simulink model "BlackBird"  (R2024b)
settings: Solver=VariableStepAuto  StartTime=0.0  StopTime=tf  RelTol=1e-3
values from neighbouring files (symbols this model uses):
  alpha0__rad = 4*pi/180    (= 0.0698131700798)    [Main.m]
  beta0__rad = 0    [Main.m]
  cbar__m = ac.cbar__m    [ComputePitchRates.m]    (also in Main.m = cbar__ft * 0.3048)
  del_ail__rad = 0.3 * pi/180    (= 0.00523598775598)    [Main.m]
  inertia_tensor = [Ixx__kgm2, 0,-Ixz__kgm2 ... (first row only)    [Main.m]
  mass__kg = mass__lb * 0.224808943    [Main.m]
  max_thrust_unit__N = max_thrust_unit__lbf * 4.448    [Main.m]
  p0__rad_s = 0    [Main.m]
  phi0__rad = 0    [Main.m]
  psi0__rad = 0    [Main.m]
  q0__rad_s = 0    [Main.m]
  r0__rad_s = 0    [Main.m]
  theta0__rad = 0    [Main.m]
  throttle = 0.1072    [Main.m]
  u0__m_s = 600    [Main.m]
  v0__m_s = 0    [Main.m]
  w0__m_s = 0    [Main.m]
  wingarea__m2 = ac.wingarea__m2    [ComputePitchRates.m]    (also in ComputeRollYawRates.m; Main.m = wingarea__ft2 * 0.09290304)
  wingspan__m = ac.wingspan__m    [ComputeRollYawRates.m]    (also in Main.m = wingspan__ft * 0.3048)
  x0__m = 0    [Main.m]
  y0__m = 0    [Main.m]
  z0__m = -20000    [Main.m]
undefined symbols (not defined in the file or in its folder): A, Blackbird, CD_f, cL0_f, cl0_m, cLalpha_f__deg, clbeta_m__deg, cLdelta_f_e__deg, cldelta_m_a__deg, cldelta_m_r__deg, clp_m__rad, cLq_f__rad, clr_m__rad, cm0_m, cmalpha_m__deg, cmdelta_m_e__deg, cmq_m__rad, cn0_m, cnbeta_m__deg, cndelta_m_a__deg, cndelta_m_r__deg, cnp_m__rad, cnr_m__rad, cY0_f, cYbeta_f__deg, cYdelta_f_a__deg, cYdelta_f_r__deg, cYp_f__rad, cYr_f__rad, Earth, WGS84
libraries: simulink_extras x25, aerolibfltsims x2, simulink x2, aerolibtransform2 x1, aerolibatmos2 x1, matrix_library x1
settings Model: Creator=alexa  LastModifiedBy=alexa
settings SolverCC: AlgebraicLoopSolver=TrustRegion
settings SFSimCC: CustomCodeUndefinedFunction=UseInterfaceOnly
settings RTWCC: GPUComputeCapability=3.5

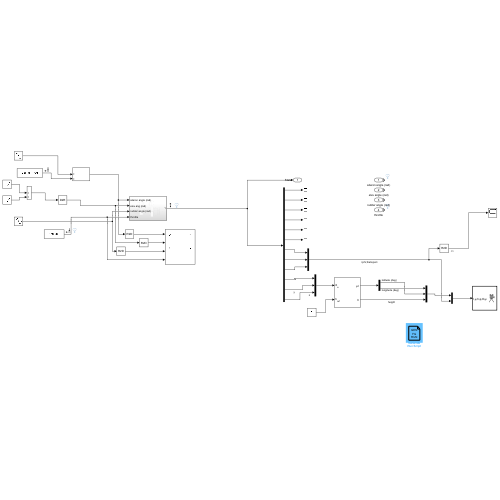
[thumbnail: Simulink's stored preview of the top-level diagram]
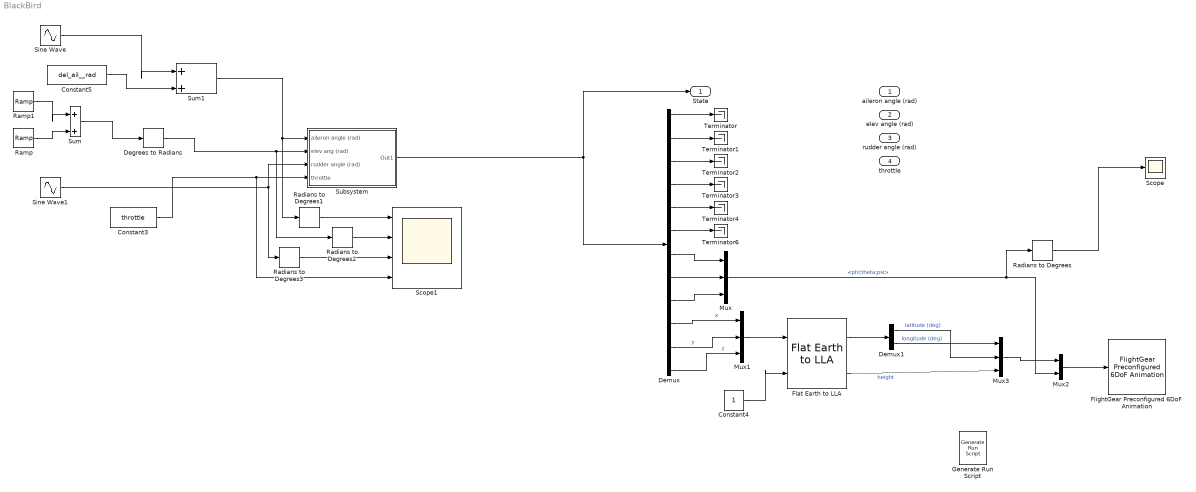
== system BlackBird ==
  aileron angle (rad) : Inport
  elev angle (rad) : Inport  Port=2
  rudder angle (rad) : Inport  Port=3
  throttle : Inport  Port=4
  Constant3 : Constant  Value=throttle
  Constant4 : Constant
  Constant5 : Constant  Value=del_ail__rad
  Degrees to Radians : simulink_extras/Transformations/Degrees to Radians
  Demux : Demux  Outputs=12
  Demux1 : Demux  Outputs=2
  Flat Earth to LLA : aerolibtransform2/Flat Earth to LLA  units=Metric (MKS)  ptype=Earth (WGS84)  F=1/298.257223563  R=6378137  refPosPort=off  LL0=[0 10]  psi=0
  FlightGear Preconfigured 6DoF Animation : aerolibfltsims/FlightGear Preconfigured 6DoF Animation  xFlightGearVersion=v2019.1  DestinationIpAddress=127.0.0.1  DestinationPort=5502  SampleTime=1/30  packetVersion=24
  Generate Run Script : aerolibfltsims/Generate Run Script  Architecture=Win64  dataFlow=Send  GeometryModelName=Blackbird-A  AirportId=KSFO  RunwayId=10L  InitialAltitude=7224  InitialHeading=113  OffsetDistance=4.72  OffsetAzimuth=0  InstallScenery=off  DisableShaders=on  OriginAddress=127.0.0.1  DestinationPort=5502  OriginPort=5505  LocalAddress=127.0.0.1  OutputFileName=runfg.bat  FlightGearBaseDirectory=C:\Program Files\FlightGear 2020.3
  Mux : Mux  Inputs=3
  Mux1 : Mux  Inputs=3
  Mux2 : Mux  Inputs=2
  Mux3 : Mux  Inputs=3
  Radians to Degrees{,1..3} (4 alike) : simulink_extras/Transformations/Radians to Degrees
  Ramp : simulink/Sources/Ramp  slope=-1  start=0  InitialOutput=0
  Ramp1 : simulink/Sources/Ramp  slope=2  start=14  InitialOutput=0
  Scope : Scope
  Scope1 : Scope  NumInputPorts=4
  Sine Wave : Sin  Amplitude=3*pi/180  Frequency=0.3  SampleTime=0
  Sine Wave1 : Sin  Amplitude=1.5*pi/180  Frequency=0.3  SampleTime=0
  Subsystem : Subsystem
  Sum : Sum  Inputs=|++
  Sum1 : Sum  Inputs=|++
  Terminator{,1..4,6} (6 alike) : Terminator
  State : Outport
  wires:
  Sum1/1 -> Radians to Degrees1/1, Subsystem/1(aileron angle (rad))
  Degrees to Radians/1 -> Radians to Degrees2/1, Subsystem/2(elev ang (rad))
  Sine Wave1/1 -> Subsystem/3(rudder angle (rad)), Radians to Degrees3/1
  Constant3/1 -> Scope1/4, Subsystem/4(throttle)
  Subsystem/1(Out1) -> Demux/1, State/1
  Demux/1 -> Terminator/1
  Demux/2 -> Terminator1/1
  Demux/3 -> Terminator2/1
  Demux/4 -> Terminator3/1
  Demux/5 -> Terminator4/1
  Demux/6 -> Terminator6/1
  Demux/7 -> Mux/1
  Demux/8 -> Mux/2
  Demux/9 -> Mux/3
  Demux/10 -> Mux1/1  "x"
  Demux/11 -> Mux1/2  "y"
  Mux/1 -> Radians to Degrees/1, Mux2/2  "<phi;theta;psi>"
  Mux2/1 -> FlightGear Preconfigured 6DoF Animation/1
  Demux/12 -> Mux1/3  "z"
  Mux1/1 -> Flat Earth to LLA/1
  Flat Earth to LLA/1 -> Demux1/1
  Demux1/1 -> Mux3/2  "latitude (deg)"
  Demux1/2 -> Mux3/1  "longitude (deg)"
  Flat Earth to LLA/2 -> Mux3/3  "height"
  Mux3/1 -> Mux2/1
  Constant4/1 -> Flat Earth to LLA/2
  Sum/1 -> Degrees to Radians/1
  Ramp/1 -> Sum/2
  Ramp1/1 -> Sum/1
  Radians to Degrees/1 -> Scope/1
  Radians to Degrees1/1 -> Scope1/1
  Radians to Degrees2/1 -> Scope1/2
  Radians to Degrees3/1 -> Scope1/3
  Sine Wave/1 -> Sum1/1
  Constant5/1 -> Sum1/2

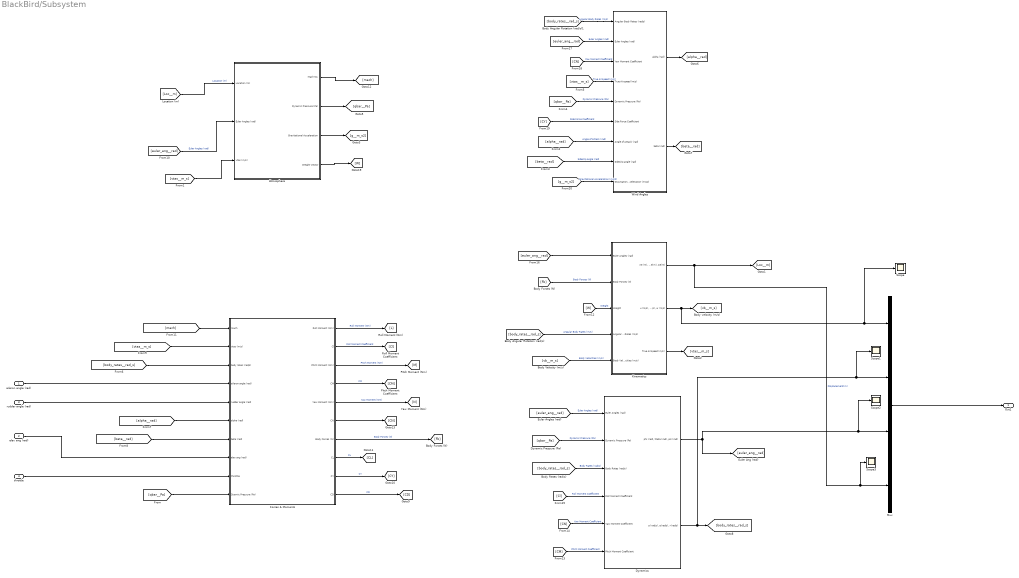
== system BlackBird/Subsystem ==
  aileron angle (rad) : Inport
  elev ang (rad) : Inport  Port=2
  rudder angle (rad) : Inport  Port=3
  throttle : Inport  Port=4
  Atmosphere : Subsystem
  Dynamics : Subsystem
  Forces & Moments : Subsystem
  Kinematics : Subsystem
  Mux : Mux
  Scope{,1..3} (4 alike) : Scope
  Wind Angles : Subsystem
  Out1 : Outport
  wires:
  Forces & Moments/9(CY) -> [CY]  "CY"
  Dynamics/2("p (rad/s), q(rad/s), r(rad/s)") -> Scope1/1, Mux/2, [body_rates__rad_s]
  [euler_ang__rad] -> Atmosphere/2(Euler Angles (rad))  "Euler Angles (rad)"
  [CM] -> Dynamics/6(Pitch Moment Coefficient)  "Pitch Moment Coefficient"
  Forces & Moments/4(CM) -> [CM]  "CM"
  [alpha__rad] -> Forces & Moments/6(alpha (rad))
  Forces & Moments/10(CD) -> [CD]  "CD"
  [mach] -> Forces & Moments/1(mach)
  [Fb] -> Kinematics/2(Body Forces (N))  "Body Forces (N)"
  Mux/1 -> Out1/1
  [W] -> Kinematics/3(Weight)  "Weight"
  Wind Angles/1(alpha (rad)) -> [alpha__rad]
  elev ang (rad)/1 -> Forces & Moments/8(elev ang (rad))
  Dynamics/1("phi (rad), theta (rad), psi (rad)") -> Scope2/1, Mux/3, [euler_ang__rad]
  [beta__rad] -> Forces & Moments/7(beta (rad))
  [euler_ang__rad] -> Wind Angles/2(Euler Angles (rad))  "Euler Angles (rad)"
  [euler_ang__rad] -> Kinematics/1(Euler Angles (rad))
  [euler_ang__rad] -> Dynamics/1(Euler Angles (rad))  "Euler Angles (rad)"
  Forces & Moments/2(Cl) -> [Cl]  "Roll Moment Coefficient"
  Kinematics/1("Xe (m), Ye(m), Ze(m)") -> [Loc__m], Scope3/1, Mux/4  "Displacement(m)"
  Forces & Moments/7(Body Forces (N)) -> [Fb]  "Body Forces (N)"
  Atmosphere/1(Mach No.) -> [mach]
  Forces & Moments/6(CN) -> [CN]
  [body_rates__rad_s] -> Forces & Moments/3(body rates (rad/s))
  [body_rates__rad_s] -> Wind Angles/1(Angular Body Rates (rad/s))  "Angular Body Rates (m/s)"
  [qbar__Pa] -> Dynamics/2(Dynamic Pressure (Pa))  "Dynamic Pressure (Pa)"
  Forces & Moments/3(Pitch Moment (Nm)) -> [M]  "Pitch Moment (Nm)"
  [vtas__m_s] -> Forces & Moments/2(vtas (m/s))
  Forces & Moments/1(Roll Moment (Nm)) -> [L]  "Roll Moment (Nm)"
  Kinematics/2("u (m/s), v(m/s), w (m/s)") -> Scope/1, Mux/1, [vb__m_s]
  Kinematics/3(True Airspeed (m/s)) -> [vtas__m_s]
  [beta__rad] -> Wind Angles/8(Sideslip angle (rad))  "Sideslip angle (rad)"
  [body_rates__rad_s] -> Dynamics/3(Body Rates (rad/s))  "Body Rates (rad/s)"
  rudder angle (rad)/1 -> Forces & Moments/5(rudder angle (rad))
  Forces & Moments/5(Yaw Moment (Nm)) -> [N]  "Yaw Moment (Nm)"
  Forces & Moments/8(CL) -> [CL]  "CL"
  [Cl] -> Dynamics/4(Roll Moment Coefficient)  "Roll Moment Coefficient"
  [CN] -> Wind Angles/3(Yaw Moment Coefficient)  "Yaw Moment Coefficient"
  Atmosphere/3(Gravitational Acceleration) -> [g__m_s2]
  [CN] -> Dynamics/5(Yaw Moment Coefficient)  "Yaw Moment Coefficient"
  [vb__m_s] -> Kinematics/5(Body Velocities (m/s))  "Body Velocities (m/s)"
  [Loc__m] -> Atmosphere/1(Location (m))  "Location (m)"
  Atmosphere/2(Dynamic Pressure (Pa)) -> [qbar__Pa]
  [qbar__Pa] -> Wind Angles/5(Dynamic Pressure (Pa))  "Dynamic Pressure (Pa)"
  Atmosphere/4(Weight Vector) -> [W]
  [body_rates__rad_s] -> Kinematics/4(Angular Body Rates (m/s))  "Angular Body Rates (m/s)"
  [alpha__rad] -> Wind Angles/7(Angle of Attack (rad))  "Angle of Attack (rad)"
  Wind Angles/2(beta (rad)) -> [beta__rad]
  [vtas__m_s] -> Wind Angles/4(True Airspeed (m/s))  "True Airspeed (m/s)"
  [g__m_s2] -> Wind Angles/9(Gravitational Acceleration (m/s2))  "Gravitational Acceleration (m/s2)"
  [CY] -> Wind Angles/6(Side Force Coefficient)  "Side Force Coefficient"
  throttle/1 -> Forces & Moments/9(throttle)
  aileron angle (rad)/1 -> Forces & Moments/4(aileron angle (rad))
  [qbar__Pa] -> Forces & Moments/10(Dyamic Pressure (Pa))
  [vtas__m_s] -> Atmosphere/3(vtas (m/s))

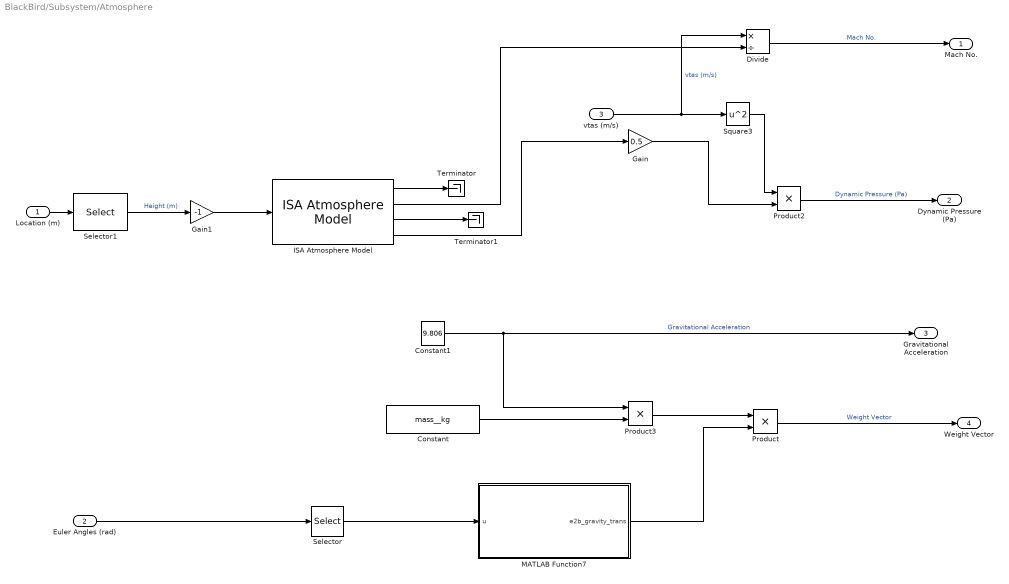
== system BlackBird/Subsystem/Atmosphere ==
  Location (m) : Inport
  Euler Angles (rad) : Inport  Port=2
  vtas (m/s) : Inport  Port=3
  Constant : Constant  Value=mass__kg
  Constant1 : Constant  Value=9.806
  Divide : Product  Inputs=*/
  Gain : Gain  Gain=0.5
  Gain1 : Gain  Gain=-1
  ISA Atmosphere Model : aerolibatmos2/ISA Atmosphere Model  useExtended=off  action=Warning  custom=off  viscosityOut=off  g=9.80665  gamma=1.4  R=287.0531  L=0.0065  h_trop=11000  h_strat=20000  rho0=1.225  P0=101325  T0=288.15  h0=0  S=110.4  Tref=273.15  muref=1.716e-5
  MATLAB Function7 : MATLAB Function  TreatAsAtomicUnit=on
  Product : Product
  Product2 : Product
  Product3 : Product
  Selector : Selector  InputPortWidth=3  IndexOptions=Index vector (dialog)  Indices=[1 2]  OutputSizes=1
  Selector1 : Selector  InputPortWidth=3  IndexOptions=Index vector (dialog)  Indices=[3]  OutputSizes=1
  Square3 : Math  Operator=square
  Terminator : Terminator
  Terminator1 : Terminator
  Mach No. : Outport
  Dynamic Pressure (Pa) : Outport  Port=2
  Gravitational Acceleration : Outport  Port=3
  Weight Vector : Outport  Port=4
  wires:
  Product3/1 -> Product/1
  ISA Atmosphere Model/1 -> Terminator/1
  Gain/1 -> Product2/2
  Constant1/1 -> Gravitational Acceleration/1, Product3/1  "Gravitational Acceleration"
  ISA Atmosphere Model/3 -> Terminator1/1
  Selector/1 -> MATLAB Function7/1(u)
  Square3/1 -> Product2/1
  ISA Atmosphere Model/4 -> Gain/1
  vtas (m/s)/1 -> Divide/1, Square3/1  "vtas (m/s)"
  MATLAB Function7/1(e2b_gravity_trans) -> Product/2
  ISA Atmosphere Model/2 -> Divide/2
  Constant/1 -> Product3/2
  Product/1 -> Weight Vector/1  "Weight Vector"
  Divide/1 -> Mach No./1  "Mach No."
  Product2/1 -> Dynamic Pressure (Pa)/1  "Dynamic Pressure (Pa)"
  Euler Angles (rad)/1 -> Selector/1
  Selector1/1 -> Gain1/1  "Height (m)"
  Location (m)/1 -> Selector1/1
  Gain1/1 -> ISA Atmosphere Model/1

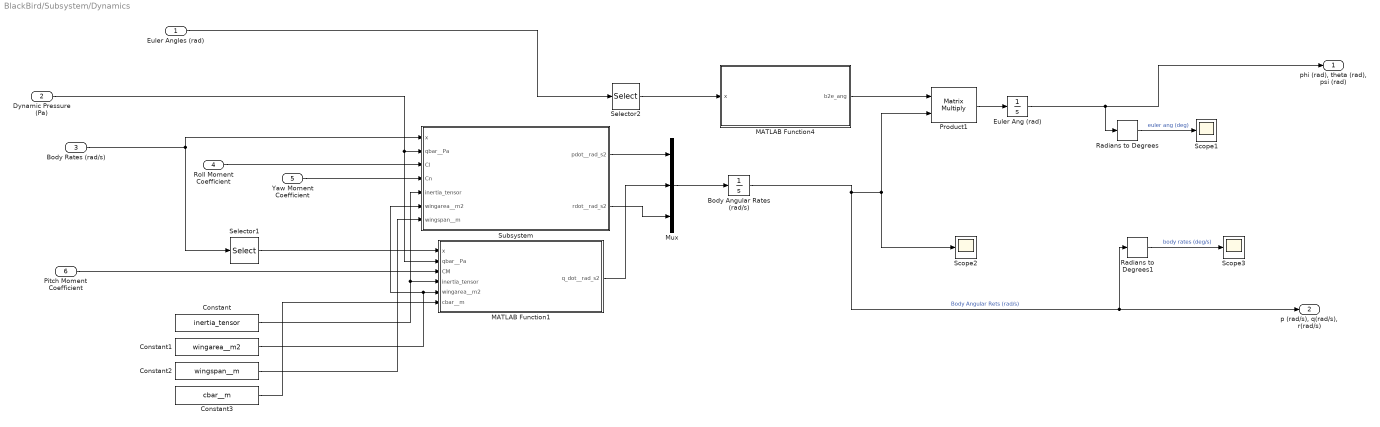
== system BlackBird/Subsystem/Dynamics ==
  Euler Angles (rad) : Inport
  Dynamic Pressure (Pa) : Inport  Port=2
  Body Rates (rad/s) : Inport  Port=3
  Roll Moment Coefficient : Inport  Port=4
  Yaw Moment Coefficient : Inport  Port=5
  Pitch Moment Coefficient : Inport  Port=6
  " Body Angular Rates (rad/s)" : Integrator  InitialCondition=[p0__rad_s;q0__rad_s;r0__rad_s]
  Constant : Constant  Value=inertia_tensor
  Constant1 : Constant  Value=wingarea__m2
  Constant2 : Constant  Value=wingspan__m
  Constant3 : Constant  Value=cbar__m
  Euler Ang (rad) : Integrator  InitialCondition=[phi0__rad;theta0__rad;psi0__rad]
  MATLAB Function1 : MATLAB Function  TreatAsAtomicUnit=on
  MATLAB Function4 : MATLAB Function  TreatAsAtomicUnit=on
  Mux : Mux  Inputs=3
  Product1 : Product  Multiplication=Matrix(*)
  Radians to Degrees : simulink_extras/Transformations/Radians to Degrees
  Radians to Degrees1 : simulink_extras/Transformations/Radians to Degrees
  Scope1 : Scope
  Scope2 : Scope
  Scope3 : Scope
  Selector1 : Selector  InputPortWidth=3  IndexOptions=Index vector (dialog)  Indices=[1 3]  OutputSizes=1
  Selector2 : Selector  InputPortWidth=3  IndexOptions=Index vector (dialog)  Indices=[1 2]  OutputSizes=1
  Subsystem : Subsystem
  "phi (rad), theta (rad), psi (rad)" : Outport
  "p (rad/s), q(rad/s), r(rad/s)" : Outport  Port=2
  wires:
  " Body Angular Rates (rad/s)"/1 -> Radians to Degrees1/1, "p (rad/s), q(rad/s), r(rad/s)"/1, Scope2/1, Product1/2  "Body Angular Rets (rad/s)"
  Dynamic Pressure (Pa)/1 -> MATLAB Function1/2(qbar__Pa), Subsystem/2(qbar__Pa)
  Selector1/1 -> MATLAB Function1/1(x)
  Product1/1 -> Euler Ang (rad)/1
  MATLAB Function4/1(b2e_ang) -> Product1/1
  Mux/1 -> " Body Angular Rates (rad/s)"/1
  Euler Ang (rad)/1 -> Radians to Degrees/1, "phi (rad), theta (rad), psi (rad)"/1
  MATLAB Function1/1(q_dot__rad_s2) -> Mux/2
  Selector2/1 -> MATLAB Function4/1(x)
  Pitch Moment Coefficient/1 -> MATLAB Function1/3(CM)
  Euler Angles (rad)/1 -> Selector2/1
  Constant/1 -> Subsystem/5(inertia_tensor), MATLAB Function1/4(inertia_tensor)
  Constant1/1 -> Subsystem/6(wingarea__m2), MATLAB Function1/5(wingarea__m2)
  Constant3/1 -> MATLAB Function1/6(cbar__m)
  Body Rates (rad/s)/1 -> Selector1/1, Subsystem/1(x)
  Roll Moment Coefficient/1 -> Subsystem/3(Cl)
  Yaw Moment Coefficient/1 -> Subsystem/4(Cn)
  Constant2/1 -> Subsystem/7(wingspan__m)
  Subsystem/1(pdot__rad_s2) -> Mux/1
  Subsystem/2(rdot__rad_s2) -> Mux/3
  Radians to Degrees/1 -> Scope1/1  "euler ang (deg)"
  Radians to Degrees1/1 -> Scope3/1  "body rates (deg/s)"

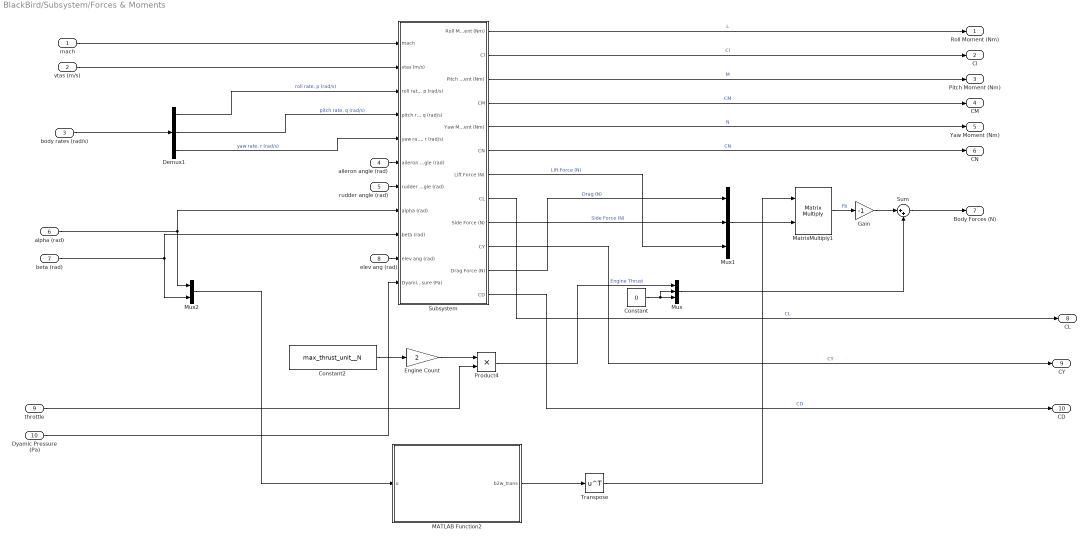
== system BlackBird/Subsystem/Forces & Moments ==
  mach : Inport
  vtas (m/s) : Inport  Port=2
  body rates (rad/s) : Inport  Port=3
  aileron angle (rad) : Inport  Port=4
  rudder angle (rad) : Inport  Port=5
  alpha (rad) : Inport  Port=6
  beta (rad) : Inport  Port=7
  elev ang (rad) : Inport  Port=8
  throttle : Inport  Port=9
  Dyamic Pressure (Pa) : Inport  Port=10
  Constant : Constant  Value=0
  Constant2 : Constant  Value=max_thrust_unit__N
  Demux1 : Demux  Outputs=3
  Engine Count : Gain  Gain=2
  Gain : Gain  Gain=-1
  MATLAB Function2 : MATLAB Function  TreatAsAtomicUnit=on
  MatrixMultiply1 : Product  Multiplication=Matrix(*)
  Mux : Mux  Inputs=3
  Mux1 : Mux  Inputs=3
  Mux2 : Mux  Inputs=2
  Product4 : Product
  Subsystem : Subsystem
  Sum : Sum  Inputs=|++
  Transpose : Math  Operator=transpose
  Roll Moment (Nm) : Outport
  Cl : Outport  Port=2
  Pitch Moment (Nm) : Outport  Port=3
  CM : Outport  Port=4
  Yaw Moment (Nm) : Outport  Port=5
  CN : Outport  Port=6
  Body Forces (N) : Outport  Port=7
  CL : Outport  Port=8
  CY : Outport  Port=9
  CD : Outport  Port=10
  wires:
  MATLAB Function2/1(b2w_trans) -> Transpose/1
  Constant2/1 -> Engine Count/1
  Transpose/1 -> MatrixMultiply1/1
  Subsystem/8(CL) -> CL/1  "CL"
  Demux1/1 -> Subsystem/3("roll rate, p (rad/s)")  "roll rate, p (rad/s)"
  throttle/1 -> Product4/2
  alpha (rad)/1 -> Mux2/1, Subsystem/8(alpha (rad))
  beta (rad)/1 -> Mux2/2, Subsystem/9(beta (rad))
  Subsystem/1(Roll Moment (Nm)) -> Roll Moment (Nm)/1  "L"
  Engine Count/1 -> Product4/1
  Subsystem/9(Side Force (N)) -> Mux1/2  "Side Force (N)"
  mach/1 -> Subsystem/1(mach)
  Mux1/1 -> MatrixMultiply1/2
  Subsystem/12(CD) -> CD/1  "CD"
  Subsystem/10(CY) -> CY/1  "CY"
  Demux1/3 -> Subsystem/5("yaw rate, r (rad/s)")  "yaw rate, r (rad/s)"
  Demux1/2 -> Subsystem/4("pitch rate, q (rad/s)")  "pitch rate, q (rad/s)"
  Subsystem/11(Drag Force (N)) -> Mux1/1  "Drag (N)"
  vtas (m/s)/1 -> Subsystem/2(vtas (m/s))
  Mux2/1 -> MATLAB Function2/1(u)
  Product4/1 -> Mux/1  "Engine Thrust"
  Subsystem/4(CM) -> CM/1  "CM"
  body rates (rad/s)/1 -> Demux1/1
  aileron angle (rad)/1 -> Subsystem/6(aileron angle (rad))
  Subsystem/3(Pitch Moment (Nm)) -> Pitch Moment (Nm)/1  "M"
  Subsystem/2(Cl) -> Cl/1  "Cl"
  rudder angle (rad)/1 -> Subsystem/7(rudder angle (rad))
  Subsystem/6(CN) -> CN/1  "CN"
  Subsystem/5(Yaw Moment (Nm)) -> Yaw Moment (Nm)/1  "N"
  elev ang (rad)/1 -> Subsystem/10(elev ang (rad))
  MatrixMultiply1/1 -> Gain/1  "Fb"
  Dyamic Pressure (Pa)/1 -> Subsystem/11(Dyamic Pressure (Pa))
  Subsystem/7(Lift Force (N)) -> Mux1/3  "Lift Force (N)"
  Gain/1 -> Sum/1
  Sum/1 -> Body Forces (N)/1
  Mux/1 -> Sum/2
  Constant/1 -> Mux/3, Mux/2

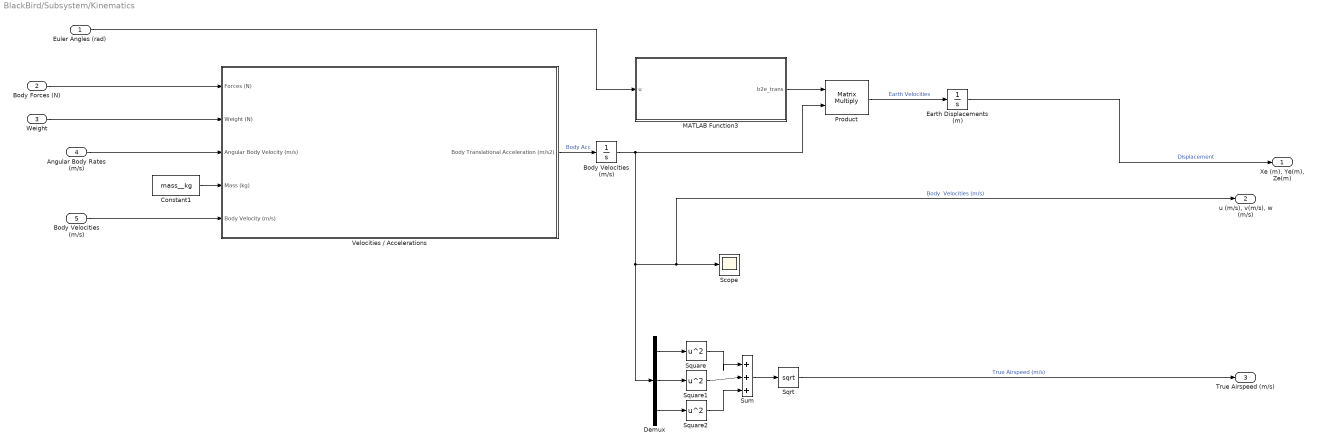
== system BlackBird/Subsystem/Kinematics ==
  Euler Angles (rad) : Inport
  Body Forces (N) : Inport  Port=2
  Weight : Inport  Port=3
  Angular Body Rates (m/s) : Inport  Port=4
  Body Velocities (m/s) : Inport  Port=5
  " Body Velocities (m/s)" : Integrator  InitialCondition=[u0__m_s;v0__m_s;w0__m_s]
  Constant1 : Constant  Value=mass__kg
  Demux : Demux  Outputs=3
  Earth Displacements (m) : Integrator  InitialCondition=[x0__m;y0__m;z0__m]
  MATLAB Function3 : MATLAB Function  TreatAsAtomicUnit=on
  Product : Product  Multiplication=Matrix(*)
  Scope : Scope
  Sqrt : Sqrt
  Square : Math  Operator=square
  Square1 : Math  Operator=square
  Square2 : Math  Operator=square
  Sum : Sum  Inputs=|+++
  Velocities / Accelerations : Subsystem
  "Xe (m), Ye(m), Ze(m)" : Outport
  "u (m/s), v(m/s), w (m/s)" : Outport  Port=2
  True Airspeed (m/s) : Outport  Port=3
  wires:
  Square1/1 -> Sum/2
  Euler Angles (rad)/1 -> MATLAB Function3/1(u)
  Square2/1 -> Sum/3
  Sum/1 -> Sqrt/1
  Square/1 -> Sum/1
  Demux/1 -> Square/1
  MATLAB Function3/1(b2e_trans) -> Product/1
  Velocities / Accelerations/1(Body Translational Acceleration (m/s2)) -> " Body Velocities (m/s)"/1  "Body Acc"
  Product/1 -> Earth Displacements (m)/1  "Earth Velocities"
  Weight/1 -> Velocities / Accelerations/2(Weight (N))
  Demux/2 -> Square1/1
  Demux/3 -> Square2/1
  Sqrt/1 -> True Airspeed (m/s)/1  "True Airspeed (m/s)"
  " Body Velocities (m/s)"/1 -> Demux/1, "u (m/s), v(m/s), w (m/s)"/1, Scope/1, Product/2  "Body  Velocities (m/s)"
  Constant1/1 -> Velocities / Accelerations/4(Mass (kg))
  Body Forces (N)/1 -> Velocities / Accelerations/1(Forces (N))
  Body Velocities (m/s)/1 -> Velocities / Accelerations/5(Body Velocity (m/s))
  Earth Displacements (m)/1 -> "Xe (m), Ye(m), Ze(m)"/1  "Displacement"
  Angular Body Rates (m/s)/1 -> Velocities / Accelerations/3(Angular Body Velocity (m/s))

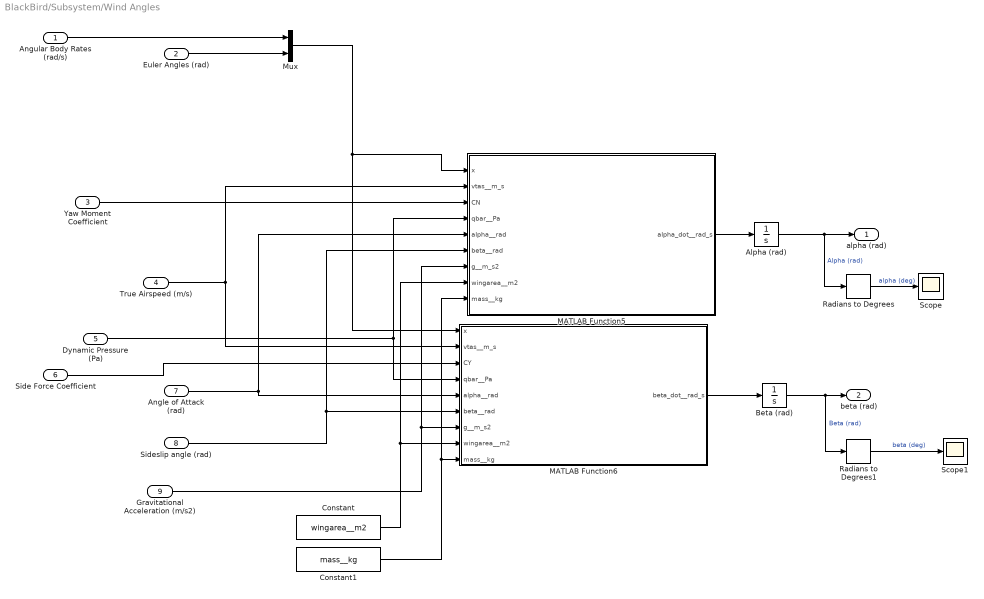
== system BlackBird/Subsystem/Wind Angles ==
  Angular Body Rates (rad/s) : Inport
  Euler Angles (rad) : Inport  Port=2
  Yaw Moment Coefficient : Inport  Port=3
  True Airspeed (m/s) : Inport  Port=4
  Dynamic Pressure (Pa) : Inport  Port=5
  Side Force Coefficient : Inport  Port=6
  Angle of Attack (rad) : Inport  Port=7
  Sideslip angle (rad) : Inport  Port=8
  Gravitational Acceleration (m/s2) : Inport  Port=9
  " Alpha (rad)" : Integrator  InitialCondition=alpha0__rad
  " Beta (rad)" : Integrator  InitialCondition=beta0__rad
  Constant : Constant  Value=wingarea__m2
  Constant1 : Constant  Value=mass__kg
  MATLAB Function5 : MATLAB Function  TreatAsAtomicUnit=on
  MATLAB Function6 : MATLAB Function  TreatAsAtomicUnit=on
  Mux : Mux  Inputs=2
  Radians to Degrees : simulink_extras/Transformations/Radians to Degrees
  Radians to Degrees1 : simulink_extras/Transformations/Radians to Degrees
  Scope : Scope
  Scope1 : Scope
  alpha (rad) : Outport
  beta (rad) : Outport  Port=2
  wires:
  Sideslip angle (rad)/1 -> MATLAB Function5/6(beta__rad), MATLAB Function6/6(beta__rad)
  MATLAB Function6/1(beta_dot__rad_s) -> " Beta (rad)"/1
  Angle of Attack (rad)/1 -> MATLAB Function5/5(alpha__rad), MATLAB Function6/5(alpha__rad)
  Dynamic Pressure (Pa)/1 -> MATLAB Function5/4(qbar__Pa), MATLAB Function6/4(qbar__Pa)
  Gravitational Acceleration (m/s2)/1 -> MATLAB Function5/7(g__m_s2), MATLAB Function6/7(g__m_s2)
  Mux/1 -> MATLAB Function6/1(x), MATLAB Function5/1(x)
  True Airspeed (m/s)/1 -> MATLAB Function5/2(vtas__m_s), MATLAB Function6/2(vtas__m_s)
  MATLAB Function5/1(alpha_dot__rad_s) -> " Alpha (rad)"/1
  Side Force Coefficient/1 -> MATLAB Function6/3(CY)
  " Alpha (rad)"/1 -> Radians to Degrees/1, alpha (rad)/1  "Alpha (rad)"
  Euler Angles (rad)/1 -> Mux/2
  " Beta (rad)"/1 -> Radians to Degrees1/1, beta (rad)/1  "Beta (rad)"
  Angular Body Rates (rad/s)/1 -> Mux/1
  Yaw Moment Coefficient/1 -> MATLAB Function5/3(CN)
  Constant1/1 -> MATLAB Function6/9(mass__kg), MATLAB Function5/9(mass__kg)
  Constant/1 -> MATLAB Function5/8(wingarea__m2), MATLAB Function6/8(wingarea__m2)
  Radians to Degrees/1 -> Scope/1  "alpha (deg)"
  Radians to Degrees1/1 -> Scope1/1  "beta (deg)"

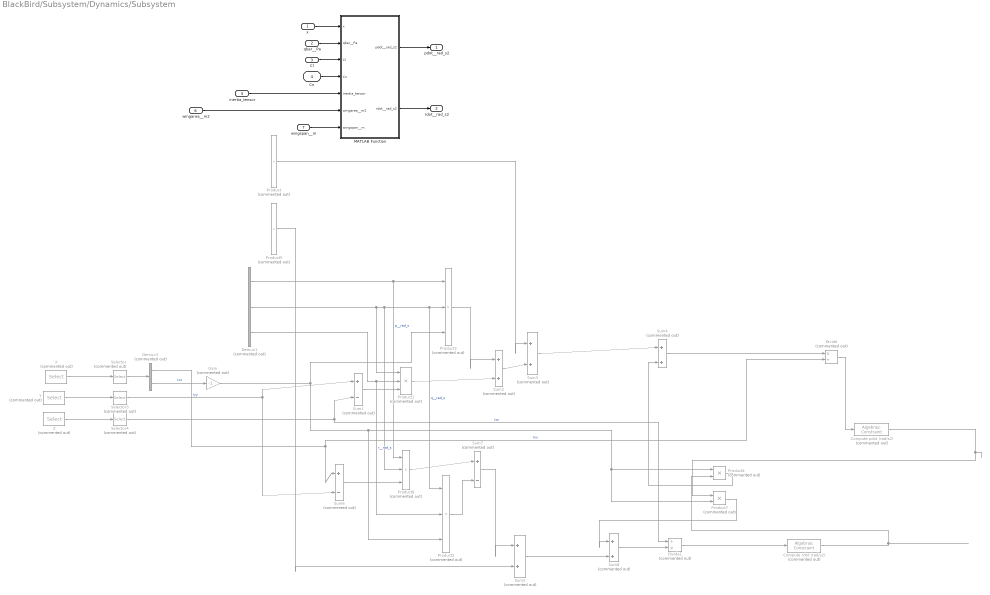
== system BlackBird/Subsystem/Dynamics/Subsystem ==
  x : Inport
  qbar__Pa : Inport  Port=2
  Cl : Inport  Port=3
  Cn : Inport  Port=4
  inertia_tensor : Inport  Port=5
  wingarea__m2 : Inport  Port=6
  wingspan__m : Inport  Port=7
  Compute pdot (rad/s2) : AlgebraicConstraint  Commented=on  Constraint=f(z) = z
  Compute rdot (rad/s2) : AlgebraicConstraint  Commented=on  Constraint=f(z) = z
  Demux1 : Demux  Commented=on  Outputs=3
  Demux3 : Demux  Commented=on  Outputs=2
  Divide : Product  Commented=on  Inputs=*/
  Divide1 : Product  Commented=on  Inputs=/*
  Gain : Gain  Commented=on  Gain=-1
  MATLAB Function : MATLAB Function  TreatAsAtomicUnit=on
  Product : Product  Commented=on  Inputs=4
  Product{1..3,6} (4 alike) : Product  Commented=on  Inputs=3
  Product4 : Product  Commented=on
  Product5 : Product  Commented=on  Inputs=4
  Product7 : Product  Commented=on
  Selector : Selector  Commented=on  InputPortWidth=3  IndexOptions=Index vector (dialog)  Indices=[1 3]  OutputSizes=1
  Selector3 : Selector  Commented=on  InputPortWidth=3  IndexOptions=Index vector (dialog)  Indices=2  OutputSizes=1
  Selector4 : Selector  Commented=on  InputPortWidth=3  IndexOptions=Index vector (dialog)  Indices=3  OutputSizes=1
  Sum1 : Sum  Commented=on  Inputs=|+-
  Sum{2..5,8} (5 alike) : Sum  Commented=on  Inputs=|++
  Sum6 : Sum  Commented=on  Inputs=|+-
  Sum7 : Sum  Commented=on  Inputs=|+-
  X : Selector  Commented=on  NumberOfDimensions=2  InputPortWidth=3  IndexOptions=Index vector (dialog),Select all  Indices=1,1  OutputSizes=1,1
  Y : Selector  Commented=on  NumberOfDimensions=2  InputPortWidth=3  IndexOptions=Index vector (dialog),Select all  Indices=2,1  OutputSizes=1,1
  Z : Selector  Commented=on  NumberOfDimensions=2  InputPortWidth=3  IndexOptions=Index vector (dialog),Select all  Indices=3,1  OutputSizes=1,1
  pdot__rad_s2 : Outport
  rdot__rad_s2 : Outport  Port=2
  wires:
  Compute pdot (rad/s2)/1 -> Product7/1
  Compute rdot (rad/s2)/1 -> Product4/2
  Selector/1 -> Demux3/1
  Selector4/1 -> Sum1/2, Divide1/1  "Izz"
  Selector3/1 -> Sum6/2, Sum1/1  "Iyy"
  Demux3/2 -> Gain/1  "Ixz"
  Demux3/1 -> Divide/2, Sum6/1  "Ixx"
  Cl/1 -> MATLAB Function/3(Cl)
  wingspan__m/1 -> MATLAB Function/7(wingspan__m)
  wingarea__m2/1 -> MATLAB Function/6(wingarea__m2)
  qbar__Pa/1 -> MATLAB Function/2(qbar__Pa)
  Sum1/1 -> Product1/3
  x/1 -> MATLAB Function/1(x)
  Demux1/3 -> Product2/2, Product1/2  "r__rad_s"
  Demux1/2 -> Product6/2, Product2/1, Product3/2, Product1/1  "q__rad_s"
  Demux1/1 -> Product6/1, Product3/1  "p__rad_s"
  Product1/1 -> Sum2/2
  Product3/1 -> Sum2/1
  Sum2/1 -> Sum3/2
  Product/1 -> Sum3/1
  Sum3/1 -> Sum4/1
  Product4/1 -> Sum4/2
  Sum4/1 -> Divide/1
  Cn/1 -> MATLAB Function/4(Cn)
  Product5/1 -> Sum5/2
  Sum6/1 -> Product6/3
  Product6/1 -> Sum7/1
  Product2/1 -> Sum7/2
  Sum7/1 -> Sum5/1
  Sum5/1 -> Sum8/2
  Product7/1 -> Sum8/1
  Sum8/1 -> Divide1/2
  Divide/1 -> Compute pdot (rad/s2)/1
  Divide1/1 -> Compute rdot (rad/s2)/1
  X/1 -> Selector/1
  Y/1 -> Selector3/1
  Z/1 -> Selector4/1
  inertia_tensor/1 -> MATLAB Function/5(inertia_tensor)
  Gain/1 -> Product3/3, Product2/3, Product7/2, Product4/1
  MATLAB Function/1(pdot__rad_s2) -> pdot__rad_s2/1
  MATLAB Function/2(rdot__rad_s2) -> rdot__rad_s2/1

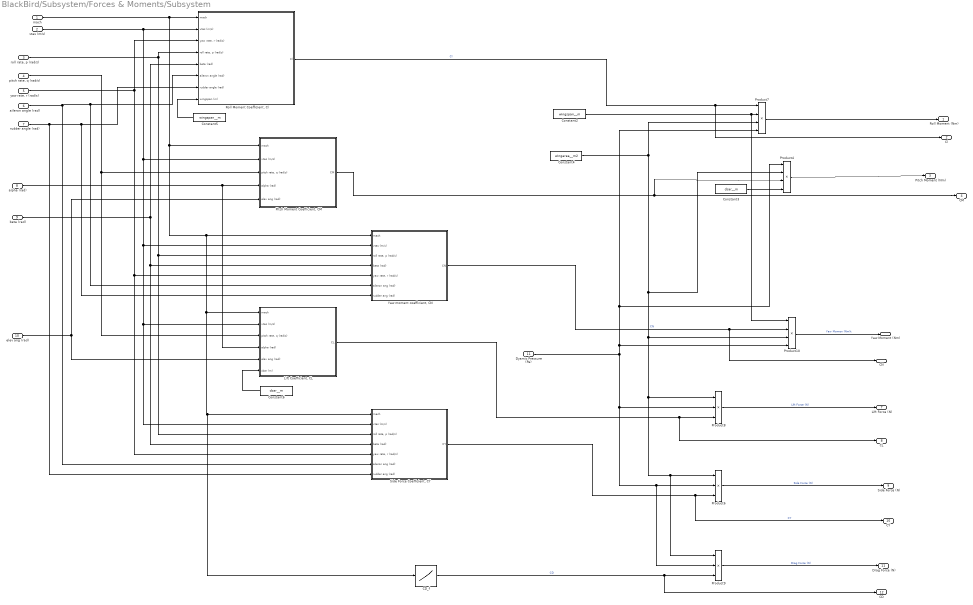
== system BlackBird/Subsystem/Forces & Moments/Subsystem ==
  mach : Inport
  vtas (m/s) : Inport  Port=2
  "roll rate, p (rad/s)" : Inport  Port=3
  "pitch rate, q (rad/s)" : Inport  Port=4
  "yaw rate, r (rad/s)" : Inport  Port=5
  aileron angle (rad) : Inport  Port=6
  rudder angle (rad) : Inport  Port=7
  alpha (rad) : Inport  Port=8
  beta (rad) : Inport  Port=9
  elev ang (rad) : Inport  Port=10
  Dyamic Pressure (Pa) : Inport  Port=11
  CD_f : Lookup_n-D  NumberOfTableDimensions=1  BreakpointsForDimension1=CD_f(:,1)  Table=CD_f(:,2)  TableMin=0.015  TableMax=0.03  InterpMethod=Cubic spline  ExtrapMethod=Clip  InternalRulePriority=Speed  RndMeth=Simplest
  Constant2 : Constant  Value=wingspan__m
  Constant3 : Constant  Value=cbar__m
  Constant4 : Constant  Value=wingarea__m2
  Constant5 : Constant  Value=wingspan__m
  Constant6 : Constant  Value=cbar__m
  "Lift Coefficient, CL" : Subsystem
  "Pitch Moment Coefficient, CM" : Subsystem
  Product10 : Product  Inputs=4
  Product4 : Product  Inputs=4
  Product6 : Product  Inputs=3
  Product7 : Product  Inputs=4
  Product8 : Product  Inputs=3
  Product9 : Product  Inputs=3
  "Roll Moment Coefficient, Cl" : Subsystem
  "Side Force Coefficient, CY" : Subsystem
  "Yaw moment coefficient, CN" : Subsystem
  Roll Moment (Nm) : Outport
  Cl : Outport  Port=2
  Pitch Moment (Nm) : Outport  Port=3
  CM : Outport  Port=4
  Yaw Moment (Nm) : Outport  Port=5
  CN : Outport  Port=6
  Lift Force (N) : Outport  Port=7
  CL : Outport  Port=8
  Side Force (N) : Outport  Port=9
  CY : Outport  Port=10
  Drag Force (N) : Outport  Port=11
  CD : Outport  Port=12
  wires:
  alpha (rad)/1 -> "Lift Coefficient, CL"/4(alpha (rad)), "Pitch Moment Coefficient, CM"/4(alpha (rad))
  Constant4/1 -> Product7/3, Product10/3, Product9/1, Product6/1, Product8/1, Product4/2
  beta (rad)/1 -> "Roll Moment Coefficient, Cl"/5(beta (rad)), "Side Force Coefficient, CY"/4(beta (rad)), "Yaw moment coefficient, CN"/4(beta (rad))
  "roll rate, p (rad/s)"/1 -> "Side Force Coefficient, CY"/3("roll rate, p (rad/s)"), "Yaw moment coefficient, CN"/3("roll rate, p (rad/s)"), "Roll Moment Coefficient, Cl"/4("roll rate, p (rad/s)")
  Constant2/1 -> Product7/2, Product10/1
  mach/1 -> "Roll Moment Coefficient, Cl"/1(mach), CD_f/1, "Side Force Coefficient, CY"/1(mach), "Lift Coefficient, CL"/1(mach), "Yaw moment coefficient, CN"/1(mach), "Pitch Moment Coefficient, CM"/1(mach)
  Constant6/1 -> "Lift Coefficient, CL"/6(cbar (m))
  CD_f/1 -> Product9/3, CD/1  "CD"
  Product10/1 -> Yaw Moment (Nm)/1  "Yaw Momen (Nm)t"
  vtas (m/s)/1 -> "Side Force Coefficient, CY"/2(vtas (m/s)), "Lift Coefficient, CL"/2(vtas (m/s)), "Yaw moment coefficient, CN"/2(vtas (m/s)), "Pitch Moment Coefficient, CM"/2(vtas (m/s)), "Roll Moment Coefficient, Cl"/2(vtas (m/s))
  Dyamic Pressure (Pa)/1 -> Product9/2, Product6/2, Product8/2, Product4/1, Product7/4, Product10/4
  "yaw rate, r (rad/s)"/1 -> "Roll Moment Coefficient, Cl"/3("yaw rate, r (rad/s)"), "Side Force Coefficient, CY"/5("yaw rate, r (rad/s)"), "Yaw moment coefficient, CN"/5("yaw rate, r (rad/s)")
  "pitch rate, q (rad/s)"/1 -> "Lift Coefficient, CL"/3("pitch rate, q (rad/s)"), "Pitch Moment Coefficient, CM"/3("pitch rate, q (rad/s)")
  "Side Force Coefficient, CY"/1(CY) -> Product6/3, CY/1  "CY"
  "Pitch Moment Coefficient, CM"/1(CM) -> CM/1, Product4/3
  "Yaw moment coefficient, CN"/1(CN) -> CN/1, Product10/2  "CN"
  Constant5/1 -> "Roll Moment Coefficient, Cl"/8(wingspan (m))
  elev ang (rad)/1 -> "Lift Coefficient, CL"/5(elev ang (rad)), "Pitch Moment Coefficient, CM"/5(elev ang (rad))
  Constant3/1 -> Product4/4
  Product4/1 -> Pitch Moment (Nm)/1
  "Roll Moment Coefficient, Cl"/1(Cl) -> Cl/1, Product7/1  "Cl"
  Product6/1 -> Side Force (N)/1  "Side Force (N)"
  "Lift Coefficient, CL"/1(CL) -> CL/1, Product8/3
  rudder angle (rad)/1 -> "Side Force Coefficient, CY"/7(rudder ang (rad)), "Yaw moment coefficient, CN"/7(rudder ang (rad)), "Roll Moment Coefficient, Cl"/7(rudder angle (rad))
  Product9/1 -> Drag Force (N)/1  "Drag Force (N)"
  aileron angle (rad)/1 -> "Yaw moment coefficient, CN"/6(aileron ang (rad)), "Roll Moment Coefficient, Cl"/6(aileron angle (rad)), "Side Force Coefficient, CY"/6(aileron ang (rad))
  Product7/1 -> Roll Moment (Nm)/1
  Product8/1 -> Lift Force (N)/1  "Lift Force (N)"

== system BlackBird/Subsystem/Kinematics/Velocities // Accelerations ==
  Forces (N) : Inport
  Weight (N) : Inport  Port=2
  Angular Body Velocity (m/s) : Inport  Port=3
  Mass (kg) : Inport  Port=4
  Body Velocity (m/s) : Inport  Port=5
  Cross Product : matrix_library/Cross Product
  Divide : Product  Inputs=*/
  Product : Product
  Sum : Sum  Inputs=|++
  Sum1 : Sum  Inputs=|+-
  Body Translational Acceleration (m/s2) : Outport
  wires:
  Forces (N)/1 -> Sum/1
  Sum1/1 -> Divide/1
  Weight (N)/1 -> Sum/2
  Sum/1 -> Sum1/1
  Product/1 -> Cross Product/2
  Angular Body Velocity (m/s)/1 -> Cross Product/1
  Mass (kg)/1 -> Divide/2, Product/1
  Cross Product/1 -> Sum1/2
  Divide/1 -> Body Translational Acceleration (m/s2)/1
  Body Velocity (m/s)/1 -> Product/2

== system BlackBird/Subsystem/Forces & Moments/Subsystem/Lift Coefficient, CL ==
  note: Inverting radian/degrees function used as
      | interp functions have angles in denominator
  mach : Inport
  vtas (m/s) : Inport  Port=2
  "pitch rate, q (rad/s)" : Inport  Port=3
  alpha (rad) : Inport  Port=4
  elev ang (rad) : Inport  Port=5
  cbar (m) : Inport  Port=6
  Divide : Product  Inputs=*/
  Gain : Gain  Gain=2
  Product : Product
  Product1 : Product  Inputs=3
  Product2 : Product
  Radians to Degrees : simulink_extras/Transformations/Radians to Degrees
  Radians to Degrees1 : simulink_extras/Transformations/Radians to Degrees
  Sum : Sum  Inputs=|++++
  cL0_f : Lookup_n-D  NumberOfTableDimensions=1  BreakpointsForDimension1=cL0_f(:,1)  Table=cL0_f(:,2)  InterpMethod=Cubic spline  ExtrapMethod=Clip  InternalRulePriority=Speed  RndMeth=Simplest
  cLalpha_f__deg : Lookup_n-D  NumberOfTableDimensions=1  BreakpointsForDimension1=cLalpha_f__deg(:,1)  Table=cLalpha_f__deg(:,2)  InterpMethod=Cubic spline  ExtrapMethod=Clip  InternalRulePriority=Speed  RndMeth=Simplest
  cLdelta_f_e__deg : Lookup_n-D  NumberOfTableDimensions=1  BreakpointsForDimension1=cLdelta_f_e__deg(:,1)  Table=cLdelta_f_e__deg(:,2)  InterpMethod=Cubic spline  ExtrapMethod=Clip  InternalRulePriority=Speed  RndMeth=Simplest
  cLq_f__rad : Lookup_n-D  NumberOfTableDimensions=1  BreakpointsForDimension1=cLq_f__rad(:,1)  Table=cLq_f__rad(:,2)  InterpMethod=Cubic spline  ExtrapMethod=Clip  InternalRulePriority=Speed  RndMeth=Simplest
  CL : Outport
  wires:
  cLalpha_f__deg/1 -> Radians to Degrees/1
  Gain/1 -> Divide/2
  mach/1 -> cLdelta_f_e__deg/1, cL0_f/1, cLalpha_f__deg/1, cLq_f__rad/1
  Product1/1 -> Sum/1
  vtas (m/s)/1 -> Gain/1
  cL0_f/1 -> Sum/3
  Divide/1 -> Product1/3
  cLdelta_f_e__deg/1 -> Radians to Degrees1/1
  Product2/1 -> Sum/4
  Product/1 -> Sum/2
  cLq_f__rad/1 -> Product1/2
  cbar (m)/1 -> Divide/1
  Sum/1 -> CL/1
  "pitch rate, q (rad/s)"/1 -> Product1/1
  elev ang (rad)/1 -> Product2/2
  alpha (rad)/1 -> Product/2
  Radians to Degrees/1 -> Product/1
  Radians to Degrees1/1 -> Product2/1

== system BlackBird/Subsystem/Forces & Moments/Subsystem/Pitch Moment Coefficient, CM ==
  note: Inverting radian/degrees function used as
      | interp functions have angles in denominator
  mach : Inport
  vtas (m/s) : Inport  Port=2
  "pitch rate, q (rad/s)" : Inport  Port=3
  alpha (rad) : Inport  Port=4
  elev ang (rad) : Inport  Port=5
  Constant : Constant  Value=cbar__m
  Divide : Product  Inputs=*/
  Gain : Gain  Gain=2
  Product : Product
  Product1 : Product  Inputs=3
  Product2 : Product
  Radians to Degrees : simulink_extras/Transformations/Radians to Degrees
  Radians to Degrees1 : simulink_extras/Transformations/Radians to Degrees
  Sum : Sum  Inputs=|++++
  cm0_m : Lookup_n-D  NumberOfTableDimensions=1  BreakpointsForDimension1=cm0_m(:,1)  Table=cm0_m(:,2)  InterpMethod=Cubic spline  ExtrapMethod=Clip  InternalRulePriority=Speed  RndMeth=Simplest
  cmalpha_m__deg : Lookup_n-D  NumberOfTableDimensions=1  BreakpointsForDimension1=cmalpha_m__deg(:,1)  Table=cmalpha_m__deg(:,2)  InterpMethod=Cubic spline  ExtrapMethod=Clip  InternalRulePriority=Speed  RndMeth=Simplest
  cmdelta_m_e__deg : Lookup_n-D  NumberOfTableDimensions=1  BreakpointsForDimension1=cmdelta_m_e__deg(:,1)  Table=cmdelta_m_e__deg(:,2)  InterpMethod=Cubic spline  ExtrapMethod=Clip  InternalRulePriority=Speed  RndMeth=Simplest
  cmq_m__rad : Lookup_n-D  NumberOfTableDimensions=1  BreakpointsForDimension1=cmq_m__rad(:,1)  Table=cmq_m__rad(:,2)  InterpMethod=Cubic spline  ExtrapMethod=Clip  InternalRulePriority=Speed  RndMeth=Simplest
  CM : Outport
  wires:
  cmalpha_m__deg/1 -> Radians to Degrees1/1
  Gain/1 -> Divide/2
  mach/1 -> cmq_m__rad/1, cmdelta_m_e__deg/1, cm0_m/1, cmalpha_m__deg/1
  Product1/1 -> Sum/1
  vtas (m/s)/1 -> Gain/1
  cm0_m/1 -> Sum/3
  Divide/1 -> Product1/3
  cmdelta_m_e__deg/1 -> Radians to Degrees/1
  Product2/1 -> Sum/4
  Product/1 -> Sum/2
  cmq_m__rad/1 -> Product1/2
  Constant/1 -> Divide/1
  Sum/1 -> CM/1
  "pitch rate, q (rad/s)"/1 -> Product1/1
  elev ang (rad)/1 -> Product2/2
  alpha (rad)/1 -> Product/2
  Radians to Degrees1/1 -> Product/1
  Radians to Degrees/1 -> Product2/1

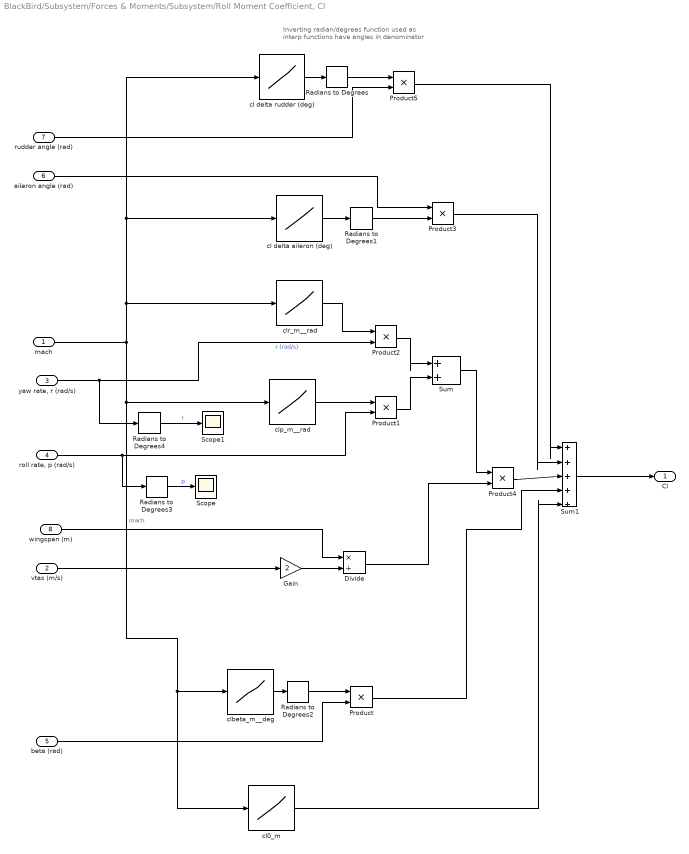
== system BlackBird/Subsystem/Forces & Moments/Subsystem/Roll Moment Coefficient, Cl ==
  note: Inverting radian/degrees function used as
      | interp functions have angles in denominator
  mach : Inport
  vtas (m/s) : Inport  Port=2
  "yaw rate, r (rad/s)" : Inport  Port=3
  "roll rate, p (rad/s)" : Inport  Port=4
  beta (rad) : Inport  Port=5
  aileron angle (rad) : Inport  Port=6
  rudder angle (rad) : Inport  Port=7
  wingspan (m) : Inport  Port=8
  Divide : Product  Inputs=*/
  Gain : Gain  Gain=2
  Product{,1..5} (6 alike) : Product
  Radians to Degrees{,1..4} (5 alike) : simulink_extras/Transformations/Radians to Degrees
  Scope : Scope
  Scope1 : Scope
  Sum : Sum  Inputs=|++
  Sum1 : Sum  Inputs=|+++++
  cl delta aileron (deg) : Lookup_n-D  NumberOfTableDimensions=1  BreakpointsForDimension1=cldelta_m_a__deg(:,1)  Table=cldelta_m_a__deg(:,2)  InterpMethod=Cubic spline  ExtrapMethod=Clip  InternalRulePriority=Speed  RndMeth=Simplest
  cl delta rudder (deg) : Lookup_n-D  NumberOfTableDimensions=1  BreakpointsForDimension1=cldelta_m_r__deg(:,1)  Table=cldelta_m_r__deg(:,2)  InterpMethod=Cubic spline  ExtrapMethod=Clip  InternalRulePriority=Speed  RndMeth=Simplest
  cl0_m : Lookup_n-D  NumberOfTableDimensions=1  BreakpointsForDimension1=cl0_m(:,1)  Table=cl0_m(:,2)  InterpMethod=Cubic spline  ExtrapMethod=Clip  InternalRulePriority=Speed  RndMeth=Simplest
  clbeta_m__deg : Lookup_n-D  NumberOfTableDimensions=1  BreakpointsForDimension1=clbeta_m__deg(:,1)  Table=clbeta_m__deg(:,2)  InterpMethod=Cubic spline  ExtrapMethod=Clip  InternalRulePriority=Speed  RndMeth=Simplest
  clp_m__rad : Lookup_n-D  NumberOfTableDimensions=1  BreakpointsForDimension1=clp_m__rad(:,1)  Table=clp_m__rad(:,2)  InterpMethod=Cubic spline  ExtrapMethod=Clip  InternalRulePriority=Speed  RndMeth=Simplest
  clr_m__rad : Lookup_n-D  NumberOfTableDimensions=1  BreakpointsForDimension1=clr_m__rad(:,1)  Table=clr_m__rad(:,2)  InterpMethod=Cubic spline  ExtrapMethod=Clip  InternalRulePriority=Speed  RndMeth=Simplest
  Cl : Outport
  wires:
  clr_m__rad/1 -> Product2/1
  Product2/1 -> Sum/1
  wingspan (m)/1 -> Divide/1
  Product5/1 -> Sum1/1
  Product1/1 -> Sum/2
  beta (rad)/1 -> Product/2
  Sum/1 -> Product4/1
  Divide/1 -> Product4/2
  Product/1 -> Sum1/4
  mach/1 -> clr_m__rad/1, cl delta aileron (deg)/1, cl delta rudder (deg)/1, clbeta_m__deg/1, cl0_m/1, clp_m__rad/1  "mach"
  Product3/1 -> Sum1/2
  clbeta_m__deg/1 -> Radians to Degrees2/1
  cl0_m/1 -> Sum1/5
  Gain/1 -> Divide/2
  cl delta aileron (deg)/1 -> Radians to Degrees1/1
  "roll rate, p (rad/s)"/1 -> Radians to Degrees3/1, Product1/2
  rudder angle (rad)/1 -> Product5/2
  cl delta rudder (deg)/1 -> Radians to Degrees/1
  Product4/1 -> Sum1/3
  vtas (m/s)/1 -> Gain/1
  clp_m__rad/1 -> Product1/1
  aileron angle (rad)/1 -> Product3/1
  "yaw rate, r (rad/s)"/1 -> Radians to Degrees4/1, Product2/2  "r (rad/s)"
  Sum1/1 -> Cl/1
  Radians to Degrees2/1 -> Product/1
  Radians to Degrees/1 -> Product5/1
  Radians to Degrees1/1 -> Product3/2
  Radians to Degrees3/1 -> Scope/1  "p"
  Radians to Degrees4/1 -> Scope1/1  "r"

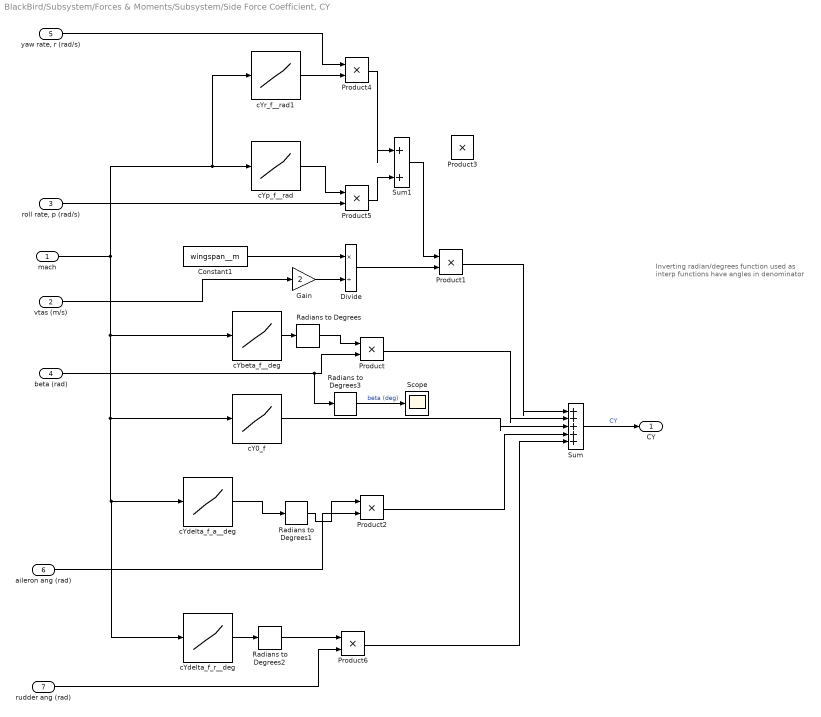
== system BlackBird/Subsystem/Forces & Moments/Subsystem/Side Force Coefficient, CY ==
  note: Inverting radian/degrees function used as
      | interp functions have angles in denominator
  mach : Inport
  vtas (m/s) : Inport  Port=2
  "roll rate, p (rad/s)" : Inport  Port=3
  beta (rad) : Inport  Port=4
  "yaw rate, r (rad/s)" : Inport  Port=5
  aileron ang (rad) : Inport  Port=6
  rudder ang (rad) : Inport  Port=7
  Constant1 : Constant  Value=wingspan__m
  Divide : Product  Inputs=*/
  Gain : Gain  Gain=2
  Product{,1..2,4..6} (6 alike) : Product
  Product3 : Product  Inputs=3
  Radians to Degrees{,1..3} (4 alike) : simulink_extras/Transformations/Radians to Degrees
  Scope : Scope
  Sum : Sum  Inputs=|+++++
  Sum1 : Sum  Inputs=|++
  cY0_f : Lookup_n-D  NumberOfTableDimensions=1  BreakpointsForDimension1=cY0_f(:,1)  Table=cY0_f(:,2)  InterpMethod=Cubic spline  ExtrapMethod=Clip  InternalRulePriority=Speed  RndMeth=Simplest
  cYbeta_f__deg : Lookup_n-D  NumberOfTableDimensions=1  BreakpointsForDimension1=cYbeta_f__deg(:,1)  Table=cYbeta_f__deg(:,2)  InterpMethod=Cubic spline  ExtrapMethod=Clip  InternalRulePriority=Speed  RndMeth=Simplest
  cYdelta_f_a__deg : Lookup_n-D  NumberOfTableDimensions=1  BreakpointsForDimension1=cYdelta_f_a__deg(:,1)  Table=cYdelta_f_a__deg(:,2)  InterpMethod=Cubic spline  ExtrapMethod=Clip  InternalRulePriority=Speed  RndMeth=Simplest
  cYdelta_f_r__deg : Lookup_n-D  NumberOfTableDimensions=1  BreakpointsForDimension1=cYdelta_f_r__deg(:,1)  Table=cYdelta_f_r__deg(:,2)  InterpMethod=Cubic spline  ExtrapMethod=Clip  InternalRulePriority=Speed  RndMeth=Simplest
  cYp_f__rad : Lookup_n-D  NumberOfTableDimensions=1  BreakpointsForDimension1=cYp_f__rad(:,1)  Table=cYp_f__rad(:,2)  InterpMethod=Cubic spline  ExtrapMethod=Clip  InternalRulePriority=Speed  RndMeth=Simplest
  cYr_f__rad1 : Lookup_n-D  NumberOfTableDimensions=1  BreakpointsForDimension1=cYr_f__rad(:,1)  Table=cYr_f__rad(:,2)  InterpMethod=Cubic spline  ExtrapMethod=Clip  InternalRulePriority=Speed  RndMeth=Simplest
  CY : Outport
  wires:
  Gain/1 -> Divide/2
  mach/1 -> cYr_f__rad1/1, cYp_f__rad/1, cYbeta_f__deg/1, cYdelta_f_r__deg/1, cYdelta_f_a__deg/1, cY0_f/1
  Product1/1 -> Sum/1
  vtas (m/s)/1 -> Gain/1
  cY0_f/1 -> Sum/3
  Divide/1 -> Product1/2
  cYdelta_f_a__deg/1 -> Radians to Degrees1/1
  Product2/1 -> Sum/4
  Product/1 -> Sum/2
  Sum1/1 -> Product1/1
  Sum/1 -> CY/1  "CY"
  aileron ang (rad)/1 -> Product2/2
  beta (rad)/1 -> Radians to Degrees3/1, Product/2
  cYbeta_f__deg/1 -> Radians to Degrees/1
  Radians to Degrees/1 -> Product/1
  Constant1/1 -> Divide/1
  cYr_f__rad1/1 -> Product4/2
  "yaw rate, r (rad/s)"/1 -> Product4/1
  "roll rate, p (rad/s)"/1 -> Product5/2
  cYp_f__rad/1 -> Product5/1
  Product5/1 -> Sum1/2
  Product4/1 -> Sum1/1
  cYdelta_f_r__deg/1 -> Radians to Degrees2/1
  rudder ang (rad)/1 -> Product6/2
  Product6/1 -> Sum/5
  Radians to Degrees1/1 -> Product2/1
  Radians to Degrees2/1 -> Product6/1
  Radians to Degrees3/1 -> Scope/1  "beta (deg)"

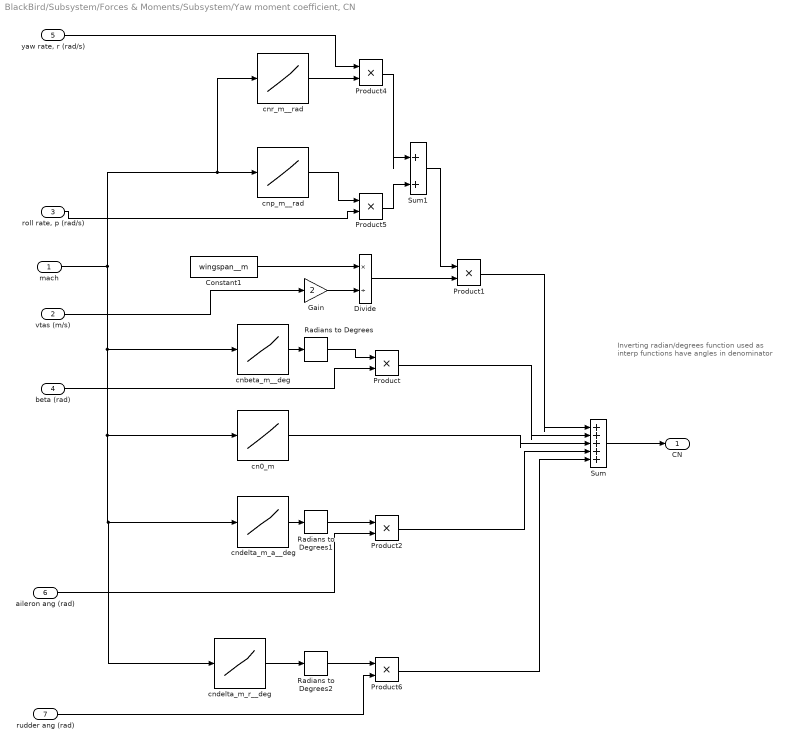
== system BlackBird/Subsystem/Forces & Moments/Subsystem/Yaw moment coefficient, CN ==
  note: Inverting radian/degrees function used as
      | interp functions have angles in denominator
  mach : Inport
  vtas (m/s) : Inport  Port=2
  "roll rate, p (rad/s)" : Inport  Port=3
  beta (rad) : Inport  Port=4
  "yaw rate, r (rad/s)" : Inport  Port=5
  aileron ang (rad) : Inport  Port=6
  rudder ang (rad) : Inport  Port=7
  Constant1 : Constant  Value=wingspan__m
  Divide : Product  Inputs=*/
  Gain : Gain  Gain=2
  Product{,1..2,4..6} (6 alike) : Product
  Radians to Degrees : simulink_extras/Transformations/Radians to Degrees
  Radians to Degrees1 : simulink_extras/Transformations/Radians to Degrees
  Radians to Degrees2 : simulink_extras/Transformations/Radians to Degrees
  Sum : Sum  Inputs=|+++++
  Sum1 : Sum  Inputs=|++
  cn0_m : Lookup_n-D  NumberOfTableDimensions=1  BreakpointsForDimension1=cn0_m(:,1)  Table=cn0_m(:,2)  InterpMethod=Cubic spline  ExtrapMethod=Clip  InternalRulePriority=Speed  RndMeth=Simplest
  cnbeta_m__deg : Lookup_n-D  NumberOfTableDimensions=1  BreakpointsForDimension1=cnbeta_m__deg(:,1)  Table=cnbeta_m__deg(:,2)  InterpMethod=Cubic spline  ExtrapMethod=Clip  InternalRulePriority=Speed  RndMeth=Simplest
  cndelta_m_a__deg : Lookup_n-D  NumberOfTableDimensions=1  BreakpointsForDimension1=cndelta_m_a__deg(:,1)  Table=cndelta_m_a__deg(:,2)  InterpMethod=Cubic spline  ExtrapMethod=Clip  InternalRulePriority=Speed  RndMeth=Simplest
  cndelta_m_r__deg : Lookup_n-D  NumberOfTableDimensions=1  BreakpointsForDimension1=cndelta_m_r__deg(:,1)  Table=cndelta_m_r__deg(:,2)  InterpMethod=Cubic spline  ExtrapMethod=Clip  InternalRulePriority=Speed  RndMeth=Simplest
  cnp_m__rad : Lookup_n-D  NumberOfTableDimensions=1  BreakpointsForDimension1=cnp_m__rad(:,1)  Table=cnp_m__rad(:,2)  InterpMethod=Cubic spline  ExtrapMethod=Clip  InternalRulePriority=Speed  RndMeth=Simplest
  cnr_m__rad : Lookup_n-D  NumberOfTableDimensions=1  BreakpointsForDimension1=cnr_m__rad(:,1)  Table=cnr_m__rad(:,2)  InterpMethod=Cubic spline  ExtrapMethod=Clip  InternalRulePriority=Speed  RndMeth=Simplest
  CN : Outport
  wires:
  Gain/1 -> Divide/2
  mach/1 -> cnp_m__rad/1, cnr_m__rad/1, cnbeta_m__deg/1, cn0_m/1, cndelta_m_r__deg/1, cndelta_m_a__deg/1
  Product1/1 -> Sum/1
  vtas (m/s)/1 -> Gain/1
  cn0_m/1 -> Sum/3
  Divide/1 -> Product1/2
  cndelta_m_a__deg/1 -> Radians to Degrees1/1
  Product2/1 -> Sum/4
  Product/1 -> Sum/2
  Sum1/1 -> Product1/1
  Sum/1 -> CN/1
  aileron ang (rad)/1 -> Product2/2
  beta (rad)/1 -> Product/2
  cnbeta_m__deg/1 -> Radians to Degrees/1
  Radians to Degrees/1 -> Product/1
  Constant1/1 -> Divide/1
  cnr_m__rad/1 -> Product4/2
  "yaw rate, r (rad/s)"/1 -> Product4/1
  "roll rate, p (rad/s)"/1 -> Product5/2
  cnp_m__rad/1 -> Product5/1
  Product5/1 -> Sum1/2
  Product4/1 -> Sum1/1
  cndelta_m_r__deg/1 -> Radians to Degrees2/1
  rudder ang (rad)/1 -> Product6/2
  Product6/1 -> Sum/5
  Radians to Degrees1/1 -> Product2/1
  Radians to Degrees2/1 -> Product6/1

== matlab function BlackBird/Subsystem/Dynamics/MATLAB Function1 ==
  data: x input; q_dot__rad_s2 output; qbar__Pa input; CM input; inertia_tensor input; wingarea__m2 input; cbar__m input
function q_dot__rad_s2  = ComputePitchRates(x,qbar__Pa,CM, inertia_tensor,wingarea__m2,cbar__m)

    % Unpack state vector
    p__rad_s = x(1);
    r__rad_s = x(2);

    % Unpack aircraft object
    Izz__kgm2 = inertia_tensor(3,3);
    Ixx__kgm2 = inertia_tensor(1,1);
    Ixz__kgm2 = -inertia_tensor(1,3);
    Iyy__kgm2 = inertia_tensor(2,2);


    % [1] Eq 2
    q_dot__rad_s2 = (qbar__Pa * wingarea__m2 * CM * cbar__m + r__rad_s * p__rad_s * (Izz__kgm2 - Ixx__kgm2) + ...
        (r__rad_s.^2 - p__rad_s.^2) * Ixz__kgm2)/ Iyy__kgm2;


end

== matlab function BlackBird/Subsystem/Dynamics/Subsystem/MATLAB Function ==
  data: x input; pdot__rad_s2 output; qbar__Pa input; Cl input; Cn input; rdot__rad_s2 output; inertia_tensor input; wingarea__m2 input; wingspan__m input
function [pdot__rad_s2,rdot__rad_s2] = ComputeRollYawRates(x,qbar__Pa,Cl,Cn,inertia_tensor,wingarea__m2,wingspan__m)


    % Unpack state vector
    p__rad_s = x(1);
    q__rad_s = x(2);
    r__rad_s = x(3);

    % Unpack aircraft object
    Izz__kgm2 = inertia_tensor(3,3);
    Ixx__kgm2 = inertia_tensor(1,1);
    Ixz__kgm2 = -inertia_tensor(1,3);
    Iyy__kgm2 = inertia_tensor(2,2);


    % vars(1) = pdot__rad_s2
    % vars(2) = rdot__rad_s2
    initialGuess = [0;0];

    fun = @(vars) ...
    [qbar__Pa * wingarea__m2 * wingspan__m * Cl + q__rad_s * r__rad_s * ( ...
                Iyy__kgm2 - Izz__kgm2) + ...
                     q__rad_s * p__rad_s* Ixz__kgm2 + vars(2) * Ixz__kgm2 - Ixx__kgm2 * vars(1);     % [1] Eq 7
    qbar__Pa * wingarea__m2 * wingspan__m * Cn + q__rad_s * p__rad_s * ( ...
                Ixx__kgm2 - Iyy__kgm2) - ...
                     q__rad_s * r__rad_s* Ixz__kgm2 + vars(1) * Ixz__kgm2 - Izz__kgm2 * vars(2)];     % [1] Eq 8


    % Use fsolve to solve the system of equations
     %options = optimoptions('levenberg-marquardt', 'Display', 'iter');
     options = optimoptions('fsolve','Display', 'iter','Algorithm','Levenberg-Marquardt');
    solution = fsolve(fun, initialGuess,options);

    % Unpack solution
    pdot__rad_s2 = solution(1);
    rdot__rad_s2 = solution(2);

end

== matlab function BlackBird/Subsystem/Forces & Moments/MATLAB Function2 ==
  data: u input; b2w_trans output
function b2w_trans  = Body2WindTransformation(u)
    % Computes the Body to Wind Axes Rotation Transformation Matrix    

    % Unpack state vector
    alpha = u(1);
    beta = u(2);
    
    % Cosine and Sine of Alpha and Beta
    c_alpha = cos(alpha);
    c_beta = cos(beta);
    s_alpha = sin(alpha);
    s_beta = sin(beta);

    % Body to Wind Axes Rotation Matrix
    b2w_trans = [c_alpha * c_beta, s_beta, s_alpha * c_beta;
        -c_alpha * s_beta, c_beta, -s_alpha * s_beta;
        -s_alpha, 0, c_alpha];

end

== matlab function BlackBird/Subsystem/Kinematics/MATLAB Function3 ==
  data: u input; b2e_trans output
function b2e_trans  = DCMTransformation(u)
    % Computes the Body to Earth Rotation Transformation Matrix 

    % Unpack state vector
    phi = u(1);
    theta = u(2);
    psi = u(3);
    
    % Cosine and Sine of Euler Angles
    c_phi = cos(phi);
    c_theta = cos(theta);
    c_psi = cos(psi);
    s_phi = sin(phi);
    s_theta = sin(theta);
    s_psi = sin(psi);
    
    % Body to Earth Rotation Transformation Matrix
    b2e_trans = [c_theta*c_psi, -c_phi*s_psi+s_phi*s_theta*c_psi, s_phi*s_psi + c_phi*s_theta*c_psi;
    c_theta*s_psi, c_phi*c_psi+s_phi*s_theta*s_psi, -s_phi*c_psi + c_phi*s_theta*s_psi;
    -s_theta, s_phi*c_theta, c_phi*c_theta];

end

== matlab function BlackBird/Subsystem/Dynamics/MATLAB Function4 ==
  data: x input; b2e_ang output
function b2e_ang  = EulerTransformation(x)
    % Computes the Body to Earth Rotation Transformation Matrix 

    % Unpack state vector
    phi = x(1);
    theta = x(2);
    
    % Cosine and Sine of Euler Angles
    c_phi = cos(phi);
    c_theta = cos(theta);
    s_phi = sin(phi);
    t_theta = tan(theta);
    
    % Body to Earth Rotation Transformation Matrix
    b2e_ang = [1, s_phi*t_theta, c_phi*t_theta;
                             0, c_phi, -s_phi;
                             0, s_phi/c_theta, c_phi/c_theta]; 

end

== matlab function BlackBird/Subsystem/Wind Angles/MATLAB Function5 ==
  data: x input; alpha_dot__rad_s output; vtas__m_s input; CN input; qbar__Pa input; alpha__rad input; beta__rad input; g__m_s2 input; wingarea__m2 input; mass__kg input
function alpha_dot__rad_s = ComputeAngleAttackDerivative(x,vtas__m_s,CN, ...
    qbar__Pa,alpha__rad,beta__rad,g__m_s2,wingarea__m2,mass__kg)

    % Unpack state variables
    p__rad_s = x(1);
    q__rad_s = x(2);
    r__rad_s = x(3);
    phi__rad = x(4);
    theta__rad = x(5);   
    
    % [1] Eq 8
    alpha_dot__rad_s = -(qbar__Pa * wingarea__m2) / ( mass__kg * vtas__m_s * cos(beta__rad)) * CN * cos(alpha__rad) + q__rad_s - ...
                          tan(beta__rad) * (p__rad_s * cos(alpha__rad) + r__rad_s * sin(alpha__rad)) + ...
                        g__m_s2 / vtas__m_s / cos(beta__rad) *( cos(phi__rad) * cos(theta__rad) * cos(alpha__rad) + sin(alpha__rad) * sin(theta__rad));
    
end

== matlab function BlackBird/Subsystem/Wind Angles/MATLAB Function6 ==
  data: x input; beta_dot__rad_s output; vtas__m_s input; CY input; qbar__Pa input; alpha__rad input; beta__rad input; g__m_s2 input; wingarea__m2 input; mass__kg input
function beta_dot__rad_s = ComputeSideSlipDerivative(x,vtas__m_s,CY, ...
    qbar__Pa,alpha__rad,beta__rad,g__m_s2, wingarea__m2,mass__kg)

    % Unpack aircraft parameters


    % Unpack state variables
    p__rad_s = x(1);
    r__rad_s = x(3);
    phi__rad = x(4);
    theta__rad = x(5);


    % [1] Eq 8
    beta_dot__rad_s = qbar__Pa * wingarea__m2 / ( mass__kg * vtas__m_s) * CY + p__rad_s * sin(alpha__rad)  - r__rad_s ...
                       *cos(alpha__rad) + g__m_s2 / vtas__m_s * (sin(phi__rad) * cos(theta__rad) ...
                       *cos(beta__rad) - sin(beta__rad) * (cos(theta__rad) * cos(phi__rad) * sin(alpha__rad) ...
                       - sin(theta__rad) * cos(alpha__rad)));
    
    
end

== matlab function BlackBird/Subsystem/Atmosphere/MATLAB Function7 ==
  data: u input; e2b_gravity_trans output
function e2b_gravity_trans  = WeightVectorTransformation(u)
    % Computes the Body to Earth Rotation Transformation Matrix for gravity

    % Unpack state vector
    phi = u(1);
    theta = u(2);
    
    % Cosine and Sine of Euler Angles
    c_phi = cos(phi);
    c_theta = cos(theta);
    s_phi = sin(phi);
    s_theta = sin(theta);
    
    % Body to Earth Rotation Transformation Matrix
    e2b_gravity_trans = [-s_theta; s_phi*c_theta; c_phi*c_theta];

end
